simulink model "mavsim_chap5"  (R2020b)
settings: Solver=ode45  StartTime=0.0  StopTime=10000  FixedStep=P.Ts/10  RelTol=1e-3  EnableMultiTasking=on
InitFcn:
  | param_chap5
values from neighbouring files (symbols this model uses):
  aileron_doublet_enable = 0    [runSim.m]
  elevator_impulse_enable = 0    [runSim.m]
  rudder_doublet_enable = 1    [runSim.m]
undefined symbols (not defined in the file or in its folder): drawAircraft, forces_moments, P, u_trim
settings Model: Creator=beard  LastModifiedBy=randa
settings DataIOCC: LimitDataPoints=on  SaveFormat=Array  SignalLoggingSaveFormat=ModelDataLogs  ReturnWorkspaceOutputs=off
settings OptimizationCC: ExpressionDepthLimit=2147483647  InitFltsAndDblsToZero=on  LifeSpan=inf
settings DebuggingCC: UnderspecifiedInitializationDetection=Classic  MergeDetectMultiDrivingBlocksExec=none  SolverPrmCheckMsg=warning  FcnCallInpInsideContextMsg=warning  StateNameClashWarn=warning  SFUnexpectedBacktrackingDiag=warning  SFNoUnconditionalDefaultTransitionDiag=warning  SFExecutionAtInitializationDiag=none  ArithmeticOperatorsInVariantConditions=warning
settings HardwareCC: ProdBitPerPointer=32  ProdBitPerSizeT=32  ProdBitPerPtrDiffT=32  ProdLargestAtomicFloat=None  ProdIntDivRoundTo=Undefined  ProdEndianess=Unspecified  ProdWordSize=32  ProdHWDeviceType=32-bit Generic
settings ModelReferenceCC: PropagateSignalLabelsOutOfModel=off
settings SFSimCC: SimUseLocalCustomCode=off  CustomCodeUndefinedFunction=UseInterfaceOnly
settings RTWCC: RTWUseLocalCustomCode=off
settings CodeAppCC: StateflowObjectComments=on
settings GRTTargetCC: TargetLangStandard=C89/C90 (ANSI)  CombineOutputUpdateFcns=off  GRTInterface=on
settings ConfigComp: CovMetricSettings=dw  CovSaveCumulativeToWorkspaceVar=on  CovSaveSingleToWorkspaceVar=on  CovExternalEMLEnable=off  CovSFcnEnable=off

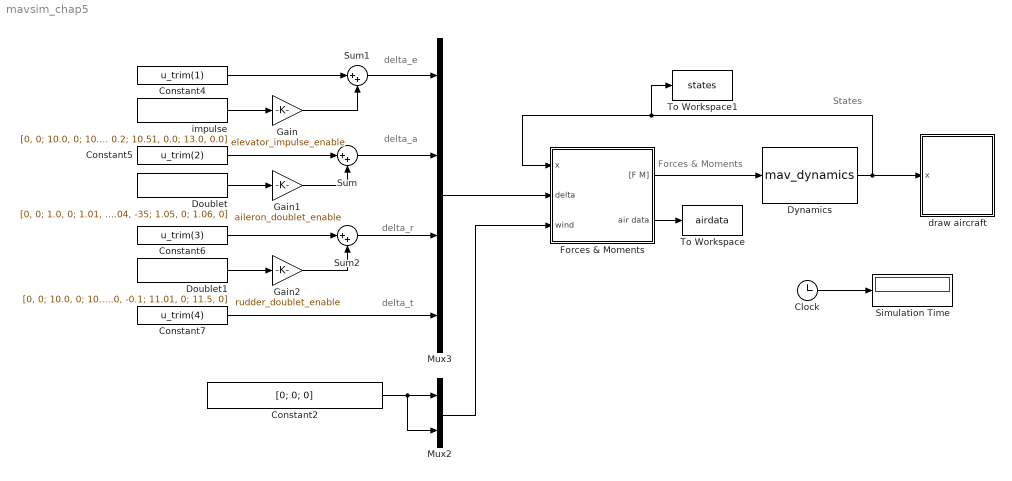
== system mavsim_chap5 ==
  note: delta_r
  note: delta_t
  note: Forces & Moments
  note: States
  note: delta_e
  note: delta_a
  Clock : Clock
  Constant2 : Constant  Value=[0; 0; 0]
  Constant4 : Constant  Value=u_trim(1)
  Constant5 : Constant  Value=u_trim(2)
  Constant6 : Constant  Value=u_trim(3)
  Constant7 : Constant  Value=u_trim(4)
  Doublet : FromWorkspace  VariableName=[0, 0; 1.0, 0; 1.01, 35; 1.02, 35; 1.03, -35; 1.04, -35; 1.05, 0; 1.06, 0]
  Doublet1 : FromWorkspace  VariableName=[0, 0; 10.0, 0; 10.01, 0.1; 10.5, 0.1; 10.51, -0.1; 11.0, -0.1; 11.01, 0; 11.5, 0]
  Dynamics : S-Function  FunctionName=mav_dynamics  Parameters=P  SFunctionDeploymentMode=off  EnableBusSupport=off
  Forces & Moments : Subsystem
  Gain : Gain  Gain=elevator_impulse_enable
  Gain1 : Gain  Gain=aileron_doublet_enable
  Gain2 : Gain  Gain=rudder_doublet_enable
  Mux2 : Mux  Inputs=2
  Mux3 : Mux
  Simulation Time : Display
  Sum : Sum  Inputs=|++
  Sum1 : Sum  Inputs=|++
  Sum2 : Sum  Inputs=|++
  To Workspace : ToWorkspace  VariableName=airdata  SaveFormat=Timeseries  SampleTime=-1
  To Workspace1 : ToWorkspace  VariableName=states  SaveFormat=Timeseries  SampleTime=-1
  draw aircraft : Subsystem
      mask Display: image(imread('tv.jpg'))
  impulse : FromWorkspace  VariableName=[0, 0; 10.0, 0; 10.01, 0.2; 10.5, 0.2; 10.51, 0.0; 13.0, 0.0]
  wires:
  Dynamics/1 -> draw aircraft/1(x), To Workspace1/1, Forces & Moments/1(x)
  Forces & Moments/1("[F M]") -> Dynamics/1
  Clock/1 -> Simulation Time/1
  Forces & Moments/2(air data) -> To Workspace/1
  Constant2/1 -> Mux2/1, Mux2/2
  Constant5/1 -> Sum/1
  Constant4/1 -> Sum1/1
  Constant6/1 -> Sum2/1
  Mux3/1 -> Forces & Moments/2(delta)
  Mux2/1 -> Forces & Moments/3(wind)
  Sum1/1 -> Mux3/1
  Sum/1 -> Mux3/2
  Sum2/1 -> Mux3/3
  Constant7/1 -> Mux3/4
  impulse/1 -> Gain/1
  Gain/1 -> Sum1/2
  Doublet/1 -> Gain1/1
  Gain1/1 -> Sum/2
  Doublet1/1 -> Gain2/1
  Gain2/1 -> Sum2/2

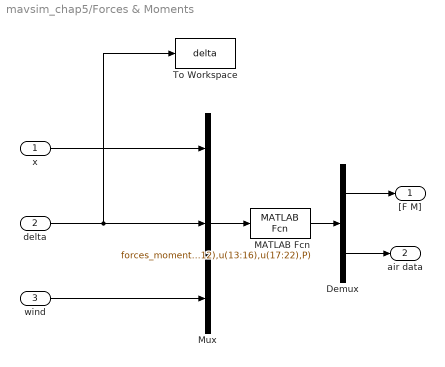
== system mavsim_chap5/Forces & Moments ==
  x : Inport
  delta : Inport  Port=2
  wind : Inport  Port=3
  Demux : Demux  Outputs=[6;6]
  MATLAB Fcn : MATLABFcn  MATLABFcn=forces_moments(u(1:12),u(13:16),u(17:22),P)  OutputDimensions=12
  Mux : Mux  Inputs=3
  To Workspace : ToWorkspace  VariableName=delta  SaveFormat=Timeseries  SampleTime=-1
  "[F M]" : Outport  VectorParamsAs1DForOutWhenUnconnected=off
  air data : Outport  Port=2  VectorParamsAs1DForOutWhenUnconnected=off
  wires:
  x/1 -> Mux/1
  delta/1 -> To Workspace/1, Mux/2
  wind/1 -> Mux/3
  MATLAB Fcn/1 -> Demux/1
  Demux/1 -> "[F M]"/1
  Mux/1 -> MATLAB Fcn/1
  Demux/2 -> air data/1

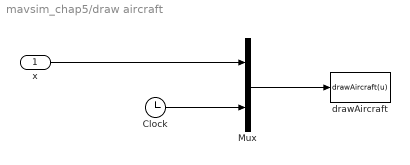
== system mavsim_chap5/draw aircraft ==
  x : Inport
  Clock : Clock
  Mux : Mux  Inputs=2
  drawAircraft : MATLABFcn  MATLABFcn=drawAircraft(u)  OutputDimensions=0  SampleTime=0.1
  wires:
  Clock/1 -> Mux/2
  x/1 -> Mux/1
  Mux/1 -> drawAircraft/1
